simulink model "MMAE_Linear_behavior_identification_with_customSignal"  (R2018b)
settings: Solver=FixedStepAuto  StartTime=0.0  StopTime=20  FixedStep=Ts_bp  RelTol=1e-3
values from neighbouring files (symbols this model uses):
  P_init = 1    [initialization.m]
  Ts = 0.1    [KinematicBicycleModel.m]    (also in LeftLaneChangeSinusoidalMotionModel.m; LinearizedBicycleModel.m; SimplifiedKinematicBicycleModel.m; amm_rel_test.m)
  Ts_bp = 0.1    [initialization.m]    (also in laneChangeSinusoidalFcn.m = 0.01; laneChangeSinusoidalJacobianFcn.m = 0.01; leftLaneChangeParametricFcn.m = 0.01; leftLaneChangeParametricWithAccFcn.m = 0.01)
  vx = X(2)    [cv_model_fun.m]    (also in initialization.m = 10)
  vy = X(4)    [cv_model_fun.m]    (also in initialization.m = 0)
  x = X(1)    [KinematicBicycleModel.m]    (also in SimplifiedKinematicBicycleModel.m; behavior_model.m = 0:0.01:20; cca_model_fun.m; ctra_model_fun.m)
  y = X(2)    [KinematicBicycleModel.m]    (also in SimplifiedKinematicBicycleModel.m; behavior_model.m = [distances velocities]; cca_model_fun.m; ctra_model_fun.m)
undefined symbols (not defined in the file or in its folder): sigbuilder_block
libraries: simulink x6
settings Model: Creator=jasprit  LastModifiedBy=jasprit
settings SFSimCC: SimUseLocalCustomCode=off
settings RTWCC: RTWUseLocalCustomCode=off

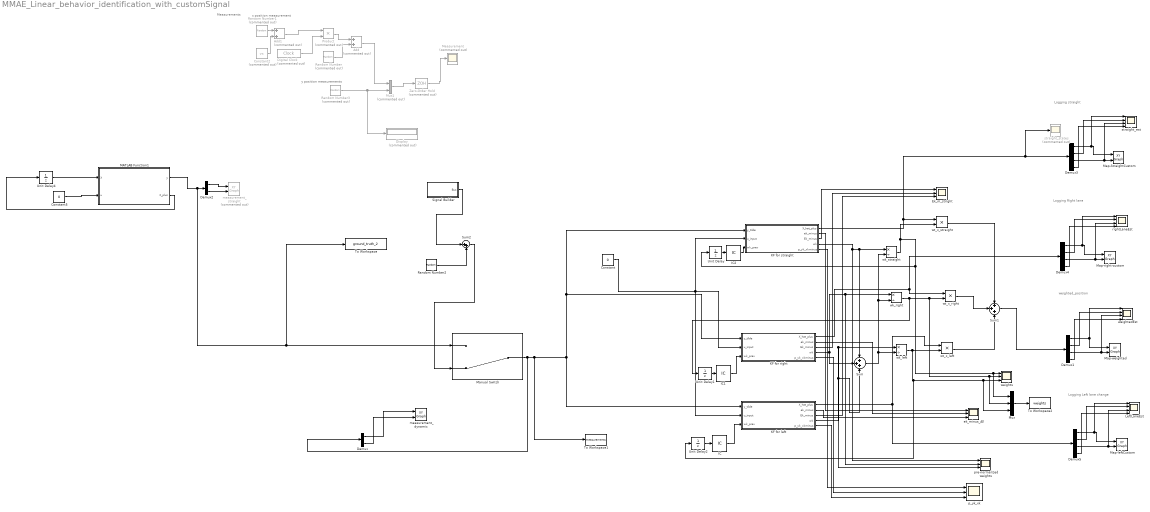
== system MMAE_Linear_behavior_identification_with_customSignal ==
  note: Logging Left lane change
  note: Logging straight
  note: Logging Right lane
  note: y position measurements
  note: x position measurement
  note: Measurements
  note: weighted_position
  Add : Sum  Commented=on
  Add1 : Sum  Commented=on
  Constant : Constant  Value=0
  Constant2 : Constant  Commented=on  Value=vx  SampleTime=Ts
  Constant5 : Constant  Value=0  SampleTime=-1
  Demux : Demux  Outputs=2
  Demux{1,3..5} (4 alike) : Demux
  Demux2 : Demux  Outputs=2
  Digital Clock : DigitalClock  Commented=on  SampleTime=Ts
  Display : Display  Commented=on
  Ek_m_stright : Scope  NumInputPorts=3
  IC : InitialCondition  Value=1/3
  IC1 : InitialCondition  Value=1/3
  IC2 : InitialCondition  Value=1/3
  "KF for left " : Subsystem
  KF for right : Subsystem
  KF for straight : Subsystem
  LeftLaneEst : Scope  NumInputPorts=4
  MATLAB Function1 : MATLAB Function  TreatAsAtomicUnit=on
  Manual Switch : ManualSwitch  CurrentSetting=0
  Map-StraightCustom : simulink/Sinks/XY Graph  xmin=-1  xmax=200  ymin=-20  ymax=20  st=-1
  Map-leftCustom : simulink/Sinks/XY Graph  xmin=-1  xmax=300  ymin=-5  ymax=5  st=-1
  Map-right-custom : simulink/Sinks/XY Graph  xmin=-1  xmax=300  ymin=-5  ymax=5  st=-1
  Map-weighted : simulink/Sinks/XY Graph  xmin=-1  xmax=300  ymin=-5  ymax=5  st=-1
  "Measurement " : Scope  Commented=on
  Mux : Mux  Inputs=3
  Mux1 : Mux  Commented=on  Inputs=2
  Product : Product  Commented=on
  Random Number : RandomNumber  Commented=on  Variance=0.0025  SampleTime=Ts
  Random Number1 : RandomNumber  Commented=on  Variance=0.0025  SampleTime=Ts
  Random Number2 : RandomNumber  Variance=0.0025  SampleTime=Ts_bp
  Random Number3 : RandomNumber  Commented=on  Variance=0.0025  SampleTime=Ts
  Signal Builder : Subsystem  Tag=STV Subsys  LoadFcn=sigbuilder_block('load');  StartFcn=sigbuilder_block('start');  StopFcn=sigbuilder_block('stop');  ClipboardFcn=sigbuilder_block('clipboard');  mask(Sigbuilder block){tuvar=[0:10]}
      mask help: Simulink:masks:SigbuilderBlock_MD
      mask init:
      | if ~strcmp(get_param(bdroot(gcbh),'SimulationStatus'),'stopped') tuvar = sigbuilder_block('maskInit'); end
      settings: CopyFcn=sigbuilder_block('copy');  DeleteFcn=sigbuilder_block('delete');  ModelCloseFcn=sigbuilder_block('modelClose');  PreSaveFcn=sigbuilder_block('preSave');  PauseFcn=sigbuilder_block('pause');  ContinueFcn=sigbuilder_block('continue');  NameChangeFcn=sigbuilder_block('namechange');  OpenFcn=sigbuilder_block('open',[552.75 8.25 565.5 444.75 ]);  CloseFcn=sigbuilder_block('close');
      mask Display: plot(0, 0, 100, 100,[2, 2, 32, 32, 2], [68, 8, 8, 68, 68],[32, 2], [38, 38], [32, 19, 2],[53, 60, 44], [32, 17, 17, 2],[16, 16, 31, 31]);txt = getActiveGroup(gcbh);text(2, 100, txt,'verticalAlignment', 'top');
  Sum : Sum  Inputs=+++
  Sum1 : Sum  Inputs=+++
  Sum2 : Sum  Inputs=|++
  To Workspace : ToWorkspace  VariableName=ground_truth_2  SaveFormat=Timeseries  SampleTime=-1
  To Workspace1 : ToWorkspace  VariableName=measurements  SaveFormat=Timeseries  SampleTime=-1
  To Workspace2 : ToWorkspace  VariableName=weights  SaveFormat=Timeseries  SampleTime=-1
  Unit Delay : UnitDelay  SampleTime=-1
  Unit Delay1 : UnitDelay  SampleTime=-1
  Unit Delay2 : UnitDelay  SampleTime=-1
  Unit Delay4 : UnitDelay  InitialCondition=[x vx y vy]  SampleTime=Ts_bp
  Zero-Order Hold : ZeroOrderHold  Commented=on  SampleTime=Ts
  ek_minus_All : Scope  NumInputPorts=3
  measurement_dynamic : simulink/Sinks/XY Graph  xmin=-1  xmax=700  ymin=-5  ymax=20  st=-1
  measurement_straight : simulink/Sinks/XY Graph  Commented=on  xmin=-1  xmax=200  ymin=-5  ymax=5  st=-1
  p_yk_xk : Scope  NumInputPorts=3
  pre-normalized weights : Scope  NumInputPorts=3
  rightLaneEst : Scope  NumInputPorts=4
  straight_est : Scope  NumInputPorts=4
  straight_states : Scope  Commented=on
  weightedEst : Scope  NumInputPorts=4
  weights : Scope  NumInputPorts=3
  wk_left : Product  Inputs=*/
  wk_right : Product  Inputs=*/
  wk_straight : Product  Inputs=*/
  wt_x_left : Product  Inputs=**
  wt_x_right : Product  Inputs=**
  wt_x_straight : Product  Inputs=**
  wires:
  Constant2/1 -> Add1/2
  Digital Clock/1 -> Product/2
  Product/1 -> Add/1
  Random Number/1 -> Add/2
  Add/1 -> Mux1/1
  Mux1/1 -> Zero-Order Hold/1
  Random Number3/1 -> Display/1, Mux1/2
  Zero-Order Hold/1 -> "Measurement "/1
  Demux3/1 -> straight_est/1, Map-StraightCustom/1
  Demux3/4 -> straight_est/4
  Demux3/2 -> straight_est/2
  Demux3/3 -> Map-StraightCustom/2, straight_est/3
  Constant/1 -> "KF for left "/2(u_input), KF for right/2(u_input), KF for straight/2(u_input)
  Demux4/1 -> rightLaneEst/1, Map-right-custom/1
  Demux4/2 -> rightLaneEst/2
  Demux4/4 -> rightLaneEst/4
  Demux4/3 -> Map-right-custom/2, rightLaneEst/3
  Demux5/1 -> LeftLaneEst/1, Map-leftCustom/1
  Demux5/4 -> LeftLaneEst/4
  Demux5/3 -> Map-leftCustom/2, LeftLaneEst/3
  Demux5/2 -> LeftLaneEst/2
  "KF for left "/1(X_hat_plus) -> wt_x_left/1, Demux5/1
  KF for right/1(X_hat_plus) -> Demux4/1, wt_x_right/1
  KF for straight/1(X_hat_plus) -> straight_states/1, Demux3/1, wt_x_straight/1
  "KF for left "/4(wk) -> pre-normalized weights/3, Sum/3, wk_left/1
  KF for right/4(wk) -> pre-normalized weights/2, wk_right/1, Sum/2
  KF for straight/4(wk) -> pre-normalized weights/1, wk_straight/1, Sum/1
  Sum/1 -> wk_left/2, wk_straight/2, wk_right/2
  wk_straight/1 -> Unit Delay/1, Mux/1, weights/1, wt_x_straight/2
  wk_right/1 -> Unit Delay1/1, Mux/2, weights/2, wt_x_right/2
  wk_left/1 -> Unit Delay2/1, Mux/3, weights/3, wt_x_left/2
  wt_x_right/1 -> Sum1/2
  wt_x_straight/1 -> Sum1/1
  wt_x_left/1 -> Sum1/3
  Demux1/1 -> weightedEst/1, Map-weighted/1
  Demux1/4 -> weightedEst/4
  Demux1/2 -> weightedEst/2
  Demux1/3 -> weightedEst/3, Map-weighted/2
  Sum1/1 -> Demux1/1
  IC2/1 -> KF for straight/3(wk_prev)
  Unit Delay/1 -> IC2/1
  IC1/1 -> KF for right/3(wk_prev)
  Unit Delay1/1 -> IC1/1
  IC/1 -> "KF for left "/3(wk_prev)
  Unit Delay2/1 -> IC/1
  KF for straight/2(ek_minus) -> ek_minus_All/1
  KF for right/2(ek_minus) -> ek_minus_All/2
  "KF for left "/2(ek_minus) -> ek_minus_All/3
  KF for straight/5(p_yk_xkminus) -> p_yk_xk/1
  KF for right/5(p_yk_xkminus) -> p_yk_xk/2
  "KF for left "/5(p_yk_xkminus) -> p_yk_xk/3
  KF for straight/3(Ek_minus) -> Ek_m_stright/1
  Manual Switch/1 -> To Workspace1/1, KF for right/1(y_tilde), KF for straight/1(y_tilde), "KF for left "/1(y_tilde), Demux/1
  Demux/1 -> measurement_dynamic/1
  Demux/2 -> measurement_dynamic/2
  MATLAB Function1/2(X_plus) -> Unit Delay4/1
  Constant5/1 -> MATLAB Function1/2(u)
  Unit Delay4/1 -> MATLAB Function1/1(X)
  MATLAB Function1/1(y) -> To Workspace/1, Manual Switch/1, Demux2/1
  Demux2/1 -> measurement_straight/1
  Demux2/2 -> measurement_straight/2
  Random Number1/1 -> Add1/1
  Add1/1 -> Product/1
  Mux/1 -> To Workspace2/1
  Signal Builder/1(Bus) -> Sum2/1
  Random Number2/1 -> Sum2/2
  Sum2/1 -> Manual Switch/2
  KF for right/3(Ek_minus) -> Ek_m_stright/2
  "KF for left "/3(Ek_minus) -> Ek_m_stright/3

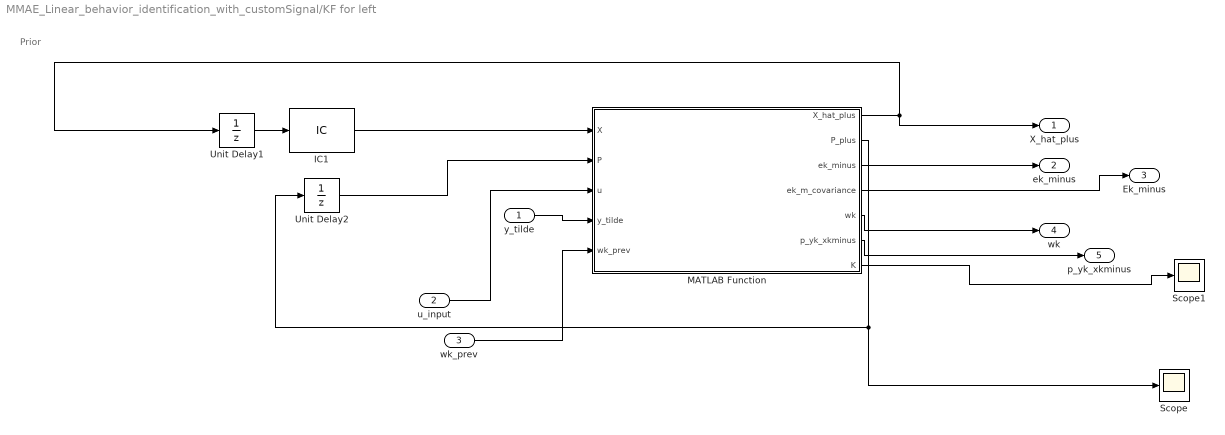
== system MMAE_Linear_behavior_identification_with_customSignal/KF for left  ==
  note: Prior
  y_tilde : Inport
  u_input : Inport  Port=2
  wk_prev : Inport  Port=3
  IC1 : InitialCondition  Value=[x vx y vy]
  MATLAB Function : MATLAB Function  TreatAsAtomicUnit=on
  Scope : Scope
  Scope1 : Scope
  Unit Delay1 : UnitDelay  SampleTime=-1
  Unit Delay2 : UnitDelay  InitialCondition=eye(4)*P_init  SampleTime=-1
  X_hat_plus : Outport
  ek_minus : Outport  Port=2
  Ek_minus : Outport  Port=3
  wk : Outport  Port=4
  p_yk_xkminus : Outport  Port=5
  wires:
  Unit Delay2/1 -> MATLAB Function/2(P)
  IC1/1 -> MATLAB Function/1(X)
  MATLAB Function/1(X_hat_plus) -> X_hat_plus/1, Unit Delay1/1
  u_input/1 -> MATLAB Function/3(u)
  Unit Delay1/1 -> IC1/1
  y_tilde/1 -> MATLAB Function/4(y_tilde)
  MATLAB Function/2(P_plus) -> Scope/1, Unit Delay2/1
  MATLAB Function/3(ek_minus) -> ek_minus/1
  MATLAB Function/4(ek_m_covariance) -> Ek_minus/1
  wk_prev/1 -> MATLAB Function/5(wk_prev)
  MATLAB Function/5(wk) -> wk/1
  MATLAB Function/6(p_yk_xkminus) -> p_yk_xkminus/1
  MATLAB Function/7(K) -> Scope1/1

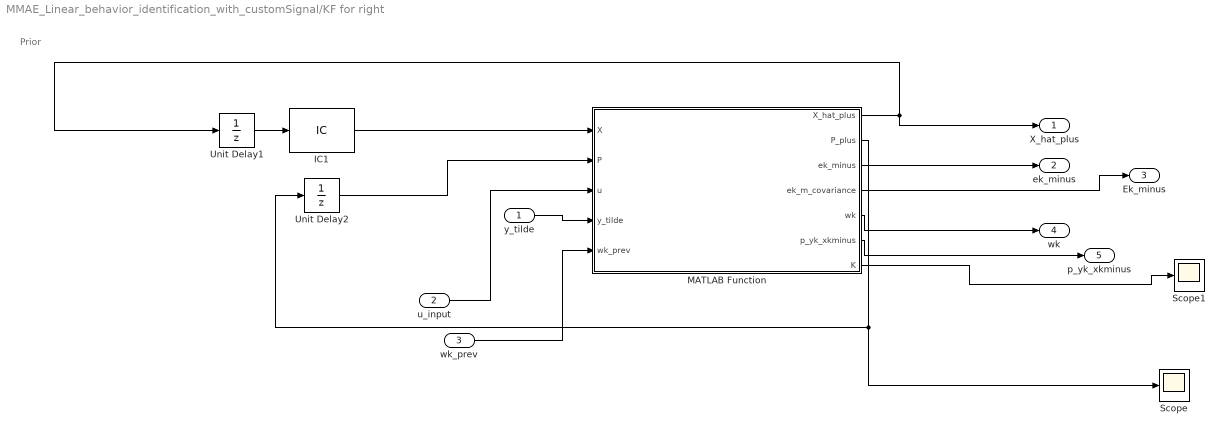
== system MMAE_Linear_behavior_identification_with_customSignal/KF for right ==
  note: Prior
  y_tilde : Inport
  u_input : Inport  Port=2
  wk_prev : Inport  Port=3
  IC1 : InitialCondition  Value=[x vx y vy]
  MATLAB Function : MATLAB Function  TreatAsAtomicUnit=on
  Scope : Scope
  Scope1 : Scope
  Unit Delay1 : UnitDelay  SampleTime=-1
  Unit Delay2 : UnitDelay  InitialCondition=eye(4)*P_init  SampleTime=-1
  X_hat_plus : Outport
  ek_minus : Outport  Port=2
  Ek_minus : Outport  Port=3
  wk : Outport  Port=4
  p_yk_xkminus : Outport  Port=5
  wires:
  Unit Delay2/1 -> MATLAB Function/2(P)
  IC1/1 -> MATLAB Function/1(X)
  MATLAB Function/1(X_hat_plus) -> X_hat_plus/1, Unit Delay1/1
  u_input/1 -> MATLAB Function/3(u)
  Unit Delay1/1 -> IC1/1
  y_tilde/1 -> MATLAB Function/4(y_tilde)
  MATLAB Function/2(P_plus) -> Scope/1, Unit Delay2/1
  MATLAB Function/3(ek_minus) -> ek_minus/1
  MATLAB Function/4(ek_m_covariance) -> Ek_minus/1
  wk_prev/1 -> MATLAB Function/5(wk_prev)
  MATLAB Function/5(wk) -> wk/1
  MATLAB Function/6(p_yk_xkminus) -> p_yk_xkminus/1
  MATLAB Function/7(K) -> Scope1/1

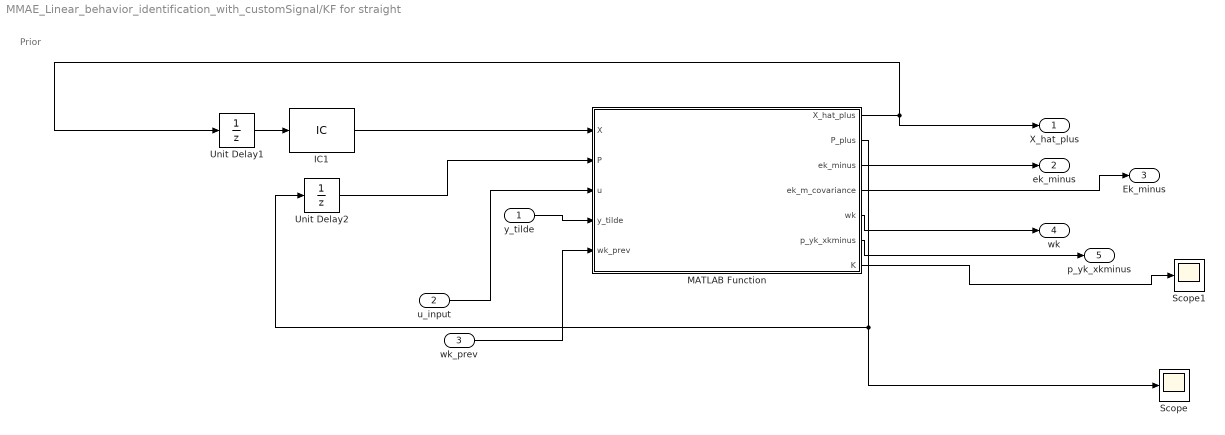
== system MMAE_Linear_behavior_identification_with_customSignal/KF for straight ==
  note: Prior
  y_tilde : Inport
  u_input : Inport  Port=2
  wk_prev : Inport  Port=3
  IC1 : InitialCondition  Value=[x vx y vy]
  MATLAB Function : MATLAB Function  TreatAsAtomicUnit=on
  Scope : Scope
  Scope1 : Scope
  Unit Delay1 : UnitDelay  SampleTime=-1
  Unit Delay2 : UnitDelay  InitialCondition=eye(4)*P_init  SampleTime=-1
  X_hat_plus : Outport
  ek_minus : Outport  Port=2
  Ek_minus : Outport  Port=3
  wk : Outport  Port=4
  p_yk_xkminus : Outport  Port=5
  wires:
  Unit Delay2/1 -> MATLAB Function/2(P)
  IC1/1 -> MATLAB Function/1(X)
  MATLAB Function/1(X_hat_plus) -> X_hat_plus/1, Unit Delay1/1
  u_input/1 -> MATLAB Function/3(u)
  Unit Delay1/1 -> IC1/1
  y_tilde/1 -> MATLAB Function/4(y_tilde)
  MATLAB Function/2(P_plus) -> Scope/1, Unit Delay2/1
  MATLAB Function/3(ek_minus) -> ek_minus/1
  MATLAB Function/4(ek_m_covariance) -> Ek_minus/1
  wk_prev/1 -> MATLAB Function/5(wk_prev)
  MATLAB Function/5(wk) -> wk/1
  MATLAB Function/6(p_yk_xkminus) -> p_yk_xkminus/1
  MATLAB Function/7(K) -> Scope1/1

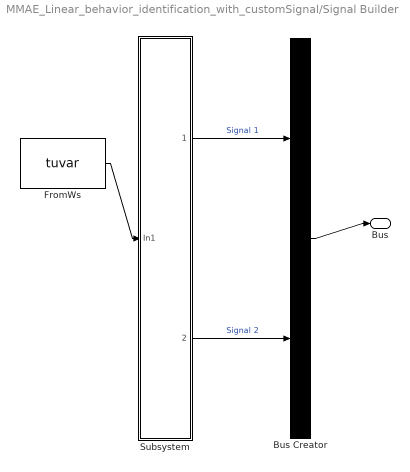
== system MMAE_Linear_behavior_identification_with_customSignal/Signal Builder ==
  Bus Creator : BusCreator  Tag=Bus Creator  Inputs=2
  FromWs : FromWorkspace  Tag=STV FromWs  VariableName=tuvar  SampleTime=0
      SigBuilderData=|
      | common.afterFinalStr = 'Extrapolate'
      | common.sampleTime = 0
      | dataSet.timeRange = [0 20]
      | dataSet.name = 'Group 1'
      | sbobj.Groups.Name = 'Group 1'
      | sbobj.Groups.Signals(1).Name = 'Signal 1'
      | sbobj.Groups.Signals(1).XData = [0 0.01 0.02 0.03 0.04 0.05 0.06 0.07 0.08 0.09 0.1 0.11 ... (2001 elements, 1x2001)]
      | sbobj.Groups.Signals(1).YData = [0 0.1 0.2 0.3 0.4 0.5 0.6 0.7 0.8 0.9 1 1.1 ... (2001 elements, 1x2001)]
      | sbobj.Groups.Signals(2).Name = 'Signal 2'
      | sbobj.Groups.Signals(2).XData = [0 0.01 0.02 0.03 0.04 0.05 0.06 0.07 0.08 0.09 0.1 0.11 ... (2001 elements, 1x2001)]
      | sbobj.Groups.Signals(2).YData = [0 0 0 0 0 0 0 0 0 0 0 0 ... (2001 elements, 1x2001)]
      | sbobj.Groups.TimeRange = [0 20]
  Subsystem : Subsystem
  Bus : Outport
  wires:
  FromWs/1 -> Subsystem/1(In1)
  Bus Creator/1 -> Bus/1
  Subsystem/1(Signal 1) -> Bus Creator/1  "Signal 1"
  Subsystem/2(Signal 2) -> Bus Creator/2  "Signal 2"

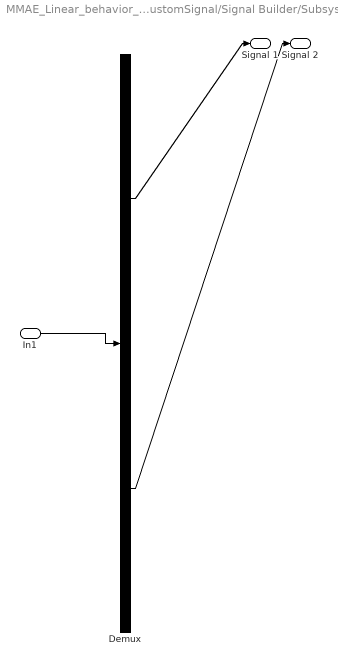
== system MMAE_Linear_behavior_identification_with_customSignal/Signal Builder/Subsystem ==
  In1 : Inport
  Demux : Demux  Tag=STV Demux  Outputs=2
  Signal 1 : Outport  Tag=STV Outport
  Signal 2 : Outport  Tag=STV Outport  Port=2
  wires:
  In1/1 -> Demux/1
  Demux/1 -> Signal 1/1
  Demux/2 -> Signal 2/1

== matlab function MMAE_Linear_behavior_identification_with_customSignal/KF for straight/MATLAB Function ==
  data: X input; P input; u input; X_hat_plus output; y_tilde input; P_plus output; ek_minus output; ek_m_covariance output; wk output; wk_prev input; p_yk_xkminus output; K output
function [X_hat_plus, P_plus, ek_minus, ek_m_covariance, wk, p_yk_xkminus, K] = kalmanFilterCustom(X, P, u, y_tilde, wk_prev)

    %%
    %TODO: See how can this be moved out of the function later
    %sampling time
    Ts_bp = 0.01;

    % measurement noise covariance
%      R = [0.25 0; 0 0.25];
   R = [0.0025 0; 0 0.0025];
    
    % process noise covariance
%     Q = diag([0.5 5.0 0.5 5.0]);
    Q = diag([0.001 0.001 0.001 0.001]);

    % states - X = [x vx y vy] - 
%     X(4) = 0;
    
    Ak = [1 Ts_bp 0 0; 0 1 0 0; 0 0 1 Ts_bp; 0 0 0 1];
%     Ak = [1 Ts_bp 0 0; 0 1 0 0; 0 0 1 Ts_bp; 0 0 0 0];
    Bk = 0;
    Ck = [1 0 0 0; 0 0 1 0];
    Dk = 0;

    %%
    % Now estimate states using kalman filter
    
    %predict
    xhat_minus = Ak * X + Bk * u;
    P_minus = (Ak * P *Ak') + Ts_bp*Q;
    yhat_minus = Ck * xhat_minus;

    %correct
    ek_minus = y_tilde - yhat_minus;    %residual
    ek_m_covariance = Ck * P_minus *Ck' + R;    %residual covariance
    K = P_minus * Ck' * inv(ek_m_covariance);
    X_hat_plus = xhat_minus + K * ek_minus;
    P_plus = (eye(4) - K * Ck) * P_minus;
    
    %calculate MMAE weights
    p_yk_xkminus = 1/sqrt(det(2*pi*ek_m_covariance))*exp(-1/2 * ek_minus'* inv(ek_m_covariance) * ek_minus);
    wk = wk_prev * p_yk_xkminus;
%       wk = p_yk_xkminus;
  
    %This will be likely outside
    %e = xhat_plus - x(:, i+1);
    
end

== matlab function MMAE_Linear_behavior_identification_with_customSignal/MATLAB Function1 ==
  data: X input; u input; y output; X_plus output
function [y, X_plus]= measurementsForStraightMotion(X, u)

    Ts_bp = 0.01;
    % states - X = [x vx y vy] -     
    Ak = [1 Ts_bp 0 0; 0 1 0 0; 0 0 1 Ts_bp; 0 0 0 1];
    Bk = 0;
    Ck = [1 0 0 0; 0 0 1 0];

    % measurement noise std_dev
%     R_sigma = [0.5 0; 0 0.5];
   R_sigma = [0.05 0; 0 0.05];
    
    % process noise std dev
%    sigma_matrix = diag([0.16 0.16 0.16 0.16]);
    sigma_matrix = diag([0.032 0.032 0.032 0.032]);
  
    X(3) = 0;
%    X(4) = 0;
    
    X_plus = Ak * X + Bk * u + sqrt(Ts_bp)*sigma_matrix*randn(4,1);    
    
    y = Ck * X_plus + R_sigma * randn(2,1);
    
end

== matlab function MMAE_Linear_behavior_identification_with_customSignal/KF for left /MATLAB Function ==
  data: X input; P input; u input; X_hat_plus output; y_tilde input; P_plus output; ek_minus output; ek_m_covariance output; wk output; wk_prev input; p_yk_xkminus output; K output
function [X_hat_plus, P_plus, ek_minus, ek_m_covariance, wk, p_yk_xkminus, K] = kalmanFilterCustom(X, P, u, y_tilde, wk_prev)

    %%
    %TODO: See how can this be moved out of the function later
    %sampling time
    Ts_bp = 0.01;

    % measurement noise covariance
%      R = [0.25 0; 0 0.25];
   R = [0.0025 0; 0 0.0025];
    
    % process noise covariance
%     Q = diag([0.5 5.0 0.5 5.0]);
    Q = diag([0.001 0.001 0.001 0.001]);

    % states - X = [x vx y vy] - 
    
%     X(4) = 0.;
    
    Ak = [1 Ts_bp 0 0; 0 1 0 0; 0 0 1 Ts_bp; 0 0 0 1];
%    Ak = [1 Ts_bp 0 0; 0 1 0 0; 0 0 1 Ts_bp; 0 0 0 1];
    Bk = 0;
    Ck = [1 0 0 0; 0 0 1 0];
    Dk = 0;

    %%
    % Now estimate states using kalman filter
    
    %predict
    xhat_minus = Ak * X + Bk * u;
    P_minus = (Ak * P *Ak') + Ts_bp*Q;
    yhat_minus = Ck * xhat_minus;

    %correct
    ek_minus = y_tilde - yhat_minus;    %residual
    ek_m_covariance = Ck * P_minus *Ck' + R;    %re20sidual covariance
    K = P_minus * Ck' * inv(ek_m_covariance);
    X_hat_plus = xhat_minus + K * ek_minus;
    P_plus = (eye(4) - K * Ck) * P_minus;
    
    %calculate MMAE weights
    p_yk_xkminus = 1/sqrt(det(2*pi*ek_m_covariance))*exp(-1/2 * ek_minus'* inv(ek_m_covariance) * ek_minus);
    wk = wk_prev * p_yk_xkminus;
%     wk = p_yk_xkminus;
    
    %This will be likely outside
    %e = xhat_plus - x(:, i+1);
    
end

== matlab function MMAE_Linear_behavior_identification_with_customSignal/KF for right/MATLAB Function ==
  data: X input; P input; u input; X_hat_plus output; y_tilde input; P_plus output; ek_minus output; ek_m_covariance output; wk output; wk_prev input; p_yk_xkminus output; K output
function [X_hat_plus, P_plus, ek_minus, ek_m_covariance, wk, p_yk_xkminus, K] = kalmanFilterCustom(X, P, u, y_tilde, wk_prev)

    %%
    %TODO: See how can this be moved out of the function later
    %sampling time
    Ts_bp = 0.01;

    % measurement noise covariance
%      R = [0.25 0; 0 0.25];
   R = [0.0025 0; 0 0.0025];
    
    % process noise covariance
%     Q = diag([0.5 5.0 0.5 5.0]);
    Q = diag([0.001 0.001 0.001 0.001]);

    % states - X = [x vx y vy] - 
%     X(4) = -0.1;
    
    Ak = [1 Ts_bp 0 0; 0 1 0 0; 0 0 1 Ts_bp; 0 0 0 1];
%     Ak = [1 Ts_bp 0 0; 0 1 0 0; 0 0 1 Ts_bp; 0 0 0 -1];
    Bk = 0;
    Ck = [1 0 0 0; 0 0 1 0];
    Dk = 0;

    %%
    % Now estimate states using kalman filter

    %predict
    xhat_minus = Ak * X + Bk * u;
%     xhat_minus(3) = -abs(xhat_minus(3));
    P_minus = (Ak * P *Ak') + Ts_bp*Q;
    yhat_minus = Ck * xhat_minus;

    %correct
    ek_minus = y_tilde - yhat_minus;    %residual
    ek_m_covariance = Ck * P_minus *Ck' + R;    %residual covariance
    K = P_minus * Ck' * inv(ek_m_covariance);
    X_hat_plus = xhat_minus + K * ek_minus;
    P_plus = (eye(4) - K * Ck) * P_minus;
    
    %calculate MMAE weights
    p_yk_xkminus = 1/sqrt(det(2*pi*ek_m_covariance))*exp(-1/2 * ek_minus'* inv(ek_m_covariance) * ek_minus);
    wk = wk_prev * p_yk_xkminus;
%     wk = p_yk_xkminus;
    
    %This will be likely outside
    %e = xhat_plus - x(:, i+1);
    
end
